simulink model "Algo_testing"  (R2017a)
settings: Solver=ode3  StartTime=0.0  StopTime=100  FixedStep=.01  RelTol=1e-3  EnableMultiTasking=on
undefined symbols (not defined in the file or in its folder): cap, soc
libraries: library x16, simulink x1
settings Model: SimulationMode=accelerator  Creator=Aniket Padghan  LastModifiedBy=Nagesh
settings DataIOCC: LimitDataPoints=on  SaveFormat=Array
settings OptimizationCC: LifeSpan=inf
settings DebuggingCC: SFUnexpectedBacktrackingDiag=warning  SFNoUnconditionalDefaultTransitionDiag=warning  SFExecutionAtInitializationDiag=none
settings HardwareCC: ProdBitPerPointer=32  ProdBitPerSizeT=32  ProdBitPerPtrDiffT=32  ProdLargestAtomicFloat=None  ProdIntDivRoundTo=Undefined  ProdEndianess=Unspecified  ProdWordSize=32  ProdHWDeviceType=32-bit Generic
settings ModelReferenceCC: PropagateSignalLabelsOutOfModel=off
settings GRTTargetCC: TargetLangStandard=C89/C90 (ANSI)  GeneratePreprocessorConditionals=Disable all
settings ConfigComp: CovMetricSettings=dw  CovHtmlReporting=on  CovSaveCumulativeToWorkspaceVar=on  CovSaveSingleToWorkspaceVar=on  CovExternalEMLEnable=off

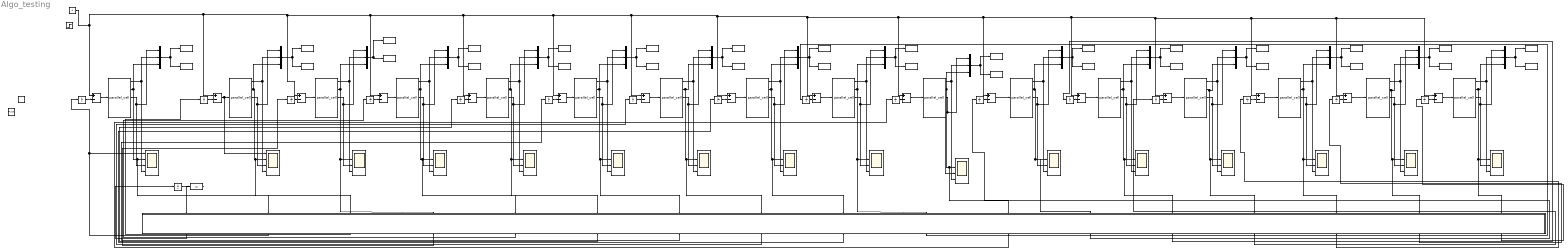
== system Algo_testing ==
  Constant : Constant  Value=-1
  IC : InitialCondition  Value=zeros(16,1)
  MATLAB Function : MATLAB Function  TreatAsAtomicUnit=on
  Mux{,1..15} (16 alike) : Mux  Inputs=3
  Pulse Generator : DiscretePulseGenerator  PulseType=Time based  Period=100  PulseWidth=50  SampleTime=0.01
  Repeating Sequence : simulink/Sources/Repeating Sequence  rep_seq_t=[0 50 100]  rep_seq_y=[0 1 0]
  Scope{,1..15} (16 alike) : Scope  NumInputPorts=4
  Step : Step  After=-1  SampleTime=0.01
  Subtract{,1,3..16} (16 alike) : Sum  Inputs=+-
  To Workspace : ToWorkspace  VariableName=VehicleBTimeSeries  SaveFormat=Timeseries  SampleTime=-1
      settings: Save2DSignal=2-D array (concatenate along first dimension)
  To Workspace1 : ToWorkspace  VariableName=VehicleBarray  SampleTime=-1
      settings: Save2DSignal=2-D array (concatenate along first dimension)
  To Workspace10 : ToWorkspace  VariableName=VehicleBTimeSeries5  SaveFormat=Timeseries  SampleTime=-1
      settings: Save2DSignal=2-D array (concatenate along first dimension)
  To Workspace11 : ToWorkspace  VariableName=VehicleBarray5  SampleTime=-1
      settings: Save2DSignal=2-D array (concatenate along first dimension)
  To Workspace12 : ToWorkspace  VariableName=VehicleBTimeSeries6  SaveFormat=Timeseries  SampleTime=-1
      settings: Save2DSignal=2-D array (concatenate along first dimension)
  To Workspace13 : ToWorkspace  VariableName=VehicleBarray6  SampleTime=-1
      settings: Save2DSignal=2-D array (concatenate along first dimension)
  To Workspace14 : ToWorkspace  VariableName=VehicleBTimeSeries7  SaveFormat=Timeseries  SampleTime=-1
      settings: Save2DSignal=2-D array (concatenate along first dimension)
  To Workspace15 : ToWorkspace  VariableName=VehicleBarray7  SampleTime=-1
      settings: Save2DSignal=2-D array (concatenate along first dimension)
  To Workspace16 : ToWorkspace  VariableName=VehicleBTimeSeries8  SaveFormat=Timeseries  SampleTime=-1
      settings: Save2DSignal=2-D array (concatenate along first dimension)
  To Workspace17 : ToWorkspace  VariableName=VehicleBarray8  SampleTime=-1
      settings: Save2DSignal=2-D array (concatenate along first dimension)
  To Workspace18 : ToWorkspace  VariableName=VehicleBTimeSeries9  SaveFormat=Timeseries  SampleTime=-1
      settings: Save2DSignal=2-D array (concatenate along first dimension)
  To Workspace19 : ToWorkspace  VariableName=VehicleBarray9  SampleTime=-1
      settings: Save2DSignal=2-D array (concatenate along first dimension)
  To Workspace2 : ToWorkspace  VariableName=VehicleBTimeSeries1  SaveFormat=Timeseries  SampleTime=-1
      settings: Save2DSignal=2-D array (concatenate along first dimension)
  To Workspace20 : ToWorkspace  VariableName=VehicleBTimeSeries10  SaveFormat=Timeseries  SampleTime=-1
      settings: Save2DSignal=2-D array (concatenate along first dimension)
  To Workspace21 : ToWorkspace  VariableName=VehicleBarray10  SampleTime=-1
      settings: Save2DSignal=2-D array (concatenate along first dimension)
  To Workspace22 : ToWorkspace  VariableName=VehicleBTimeSeries11  SaveFormat=Timeseries  SampleTime=-1
      settings: Save2DSignal=2-D array (concatenate along first dimension)
  To Workspace23 : ToWorkspace  VariableName=VehicleBarray11  SampleTime=-1
      settings: Save2DSignal=2-D array (concatenate along first dimension)
  To Workspace24 : ToWorkspace  VariableName=VehicleBTimeSeries12  SaveFormat=Timeseries  SampleTime=-1
      settings: Save2DSignal=2-D array (concatenate along first dimension)
  To Workspace25 : ToWorkspace  VariableName=VehicleBarray12  SampleTime=-1
      settings: Save2DSignal=2-D array (concatenate along first dimension)
  To Workspace26 : ToWorkspace  VariableName=VehicleBTimeSeries13  SaveFormat=Timeseries  SampleTime=-1
      settings: Save2DSignal=2-D array (concatenate along first dimension)
  To Workspace27 : ToWorkspace  VariableName=VehicleBarray13  SampleTime=-1
      settings: Save2DSignal=2-D array (concatenate along first dimension)
  To Workspace28 : ToWorkspace  VariableName=VehicleBTimeSeries14  SaveFormat=Timeseries  SampleTime=-1
      settings: Save2DSignal=2-D array (concatenate along first dimension)
  To Workspace29 : ToWorkspace  VariableName=VehicleBarray14  SampleTime=-1
      settings: Save2DSignal=2-D array (concatenate along first dimension)
  To Workspace3 : ToWorkspace  VariableName=VehicleBarray1  SampleTime=-1
      settings: Save2DSignal=2-D array (concatenate along first dimension)
  To Workspace30 : ToWorkspace  VariableName=VehicleBTimeSeries15  SaveFormat=Timeseries  SampleTime=-1
      settings: Save2DSignal=2-D array (concatenate along first dimension)
  To Workspace31 : ToWorkspace  VariableName=VehicleBarray15  SampleTime=-1
      settings: Save2DSignal=2-D array (concatenate along first dimension)
  To Workspace4 : ToWorkspace  VariableName=VehicleBTimeSeries2  SaveFormat=Timeseries  SampleTime=-1
      settings: Save2DSignal=2-D array (concatenate along first dimension)
  To Workspace5 : ToWorkspace  VariableName=VehicleBarray2  SampleTime=-1
      settings: Save2DSignal=2-D array (concatenate along first dimension)
  To Workspace6 : ToWorkspace  VariableName=VehicleBTimeSeries3  SaveFormat=Timeseries  SampleTime=-1
      settings: Save2DSignal=2-D array (concatenate along first dimension)
  To Workspace7 : ToWorkspace  VariableName=VehicleBarray3  SampleTime=-1
      settings: Save2DSignal=2-D array (concatenate along first dimension)
  To Workspace8 : ToWorkspace  VariableName=VehicleBTimeSeries4  SaveFormat=Timeseries  SampleTime=-1
      settings: Save2DSignal=2-D array (concatenate along first dimension)
  To Workspace9 : ToWorkspace  VariableName=VehicleBarray4  SampleTime=-1
      settings: Save2DSignal=2-D array (concatenate along first dimension)
  Unit Delay{,1..16} (17 alike) : UnitDelay  SampleTime=-1
  parallel_cell : library/parallel_cell  initial_SoC=soc(1)  cell_capacity=cap(1)  T_SoC_Breakpoints=T_SoC_Breakpoints  T_SoC_Table_Data=T_SoC_Table_Data  Rp_SoC_Table_Data=Rp_SoC_Table_Data  Rp_SoC_Breakpoints=Rp_SoC_Breakpoints  Ro_SoC_Table_Data=Ro_SoC_Table_Data  Ro_SoC_Breakpoints=Ro_SoC_Breakpoints  Em_SoC_Table_Data=Em_SoC_Table_Data  Em_SoC_Breakpoints=Em_SoC_Breakpoints
      link override Integrator: LowerSaturationLimit=-1*cell_capacity*3600
  parallel_cell1 : library/parallel_cell  initial_SoC=soc(2)  cell_capacity=cap(2)  T_SoC_Breakpoints=T_SoC_Breakpoints  T_SoC_Table_Data=T_SoC_Table_Data  Rp_SoC_Table_Data=Rp_SoC_Table_Data  Rp_SoC_Breakpoints=Rp_SoC_Breakpoints  Ro_SoC_Table_Data=Ro_SoC_Table_Data  Ro_SoC_Breakpoints=Ro_SoC_Breakpoints  Em_SoC_Table_Data=Em_SoC_Table_Data  Em_SoC_Breakpoints=Em_SoC_Breakpoints
      link override Integrator: LowerSaturationLimit=-1*cell_capacity*3600
  parallel_cell10 : library/parallel_cell  initial_SoC=soc(11)  cell_capacity=cap(11)  T_SoC_Breakpoints=T_SoC_Breakpoints  T_SoC_Table_Data=T_SoC_Table_Data  Rp_SoC_Table_Data=Rp_SoC_Table_Data  Rp_SoC_Breakpoints=Rp_SoC_Breakpoints  Ro_SoC_Table_Data=Ro_SoC_Table_Data  Ro_SoC_Breakpoints=Ro_SoC_Breakpoints  Em_SoC_Table_Data=Em_SoC_Table_Data  Em_SoC_Breakpoints=Em_SoC_Breakpoints
      link override Integrator: LowerSaturationLimit=-1*cell_capacity*3600
  parallel_cell11 : library/parallel_cell  initial_SoC=soc(12)  cell_capacity=cap(12)  T_SoC_Breakpoints=T_SoC_Breakpoints  T_SoC_Table_Data=T_SoC_Table_Data  Rp_SoC_Table_Data=Rp_SoC_Table_Data  Rp_SoC_Breakpoints=Rp_SoC_Breakpoints  Ro_SoC_Table_Data=Ro_SoC_Table_Data  Ro_SoC_Breakpoints=Ro_SoC_Breakpoints  Em_SoC_Table_Data=Em_SoC_Table_Data  Em_SoC_Breakpoints=Em_SoC_Breakpoints
      link override Integrator: LowerSaturationLimit=-1*cell_capacity*3600
  parallel_cell12 : library/parallel_cell  initial_SoC=soc(13)  cell_capacity=cap(13)  T_SoC_Breakpoints=T_SoC_Breakpoints  T_SoC_Table_Data=T_SoC_Table_Data  Rp_SoC_Table_Data=Rp_SoC_Table_Data  Rp_SoC_Breakpoints=Rp_SoC_Breakpoints  Ro_SoC_Table_Data=Ro_SoC_Table_Data  Ro_SoC_Breakpoints=Ro_SoC_Breakpoints  Em_SoC_Table_Data=Em_SoC_Table_Data  Em_SoC_Breakpoints=Em_SoC_Breakpoints
      link override Integrator: LowerSaturationLimit=-1*cell_capacity*3600
  parallel_cell13 : library/parallel_cell  initial_SoC=soc(14)  cell_capacity=cap(14)  T_SoC_Breakpoints=T_SoC_Breakpoints  T_SoC_Table_Data=T_SoC_Table_Data  Rp_SoC_Table_Data=Rp_SoC_Table_Data  Rp_SoC_Breakpoints=Rp_SoC_Breakpoints  Ro_SoC_Table_Data=Ro_SoC_Table_Data  Ro_SoC_Breakpoints=Ro_SoC_Breakpoints  Em_SoC_Table_Data=Em_SoC_Table_Data  Em_SoC_Breakpoints=Em_SoC_Breakpoints
      link override Integrator: LowerSaturationLimit=-1*cell_capacity*3600
  parallel_cell14 : library/parallel_cell  initial_SoC=soc(15)  cell_capacity=cap(15)  T_SoC_Breakpoints=T_SoC_Breakpoints  T_SoC_Table_Data=T_SoC_Table_Data  Rp_SoC_Table_Data=Rp_SoC_Table_Data  Rp_SoC_Breakpoints=Rp_SoC_Breakpoints  Ro_SoC_Table_Data=Ro_SoC_Table_Data  Ro_SoC_Breakpoints=Ro_SoC_Breakpoints  Em_SoC_Table_Data=Em_SoC_Table_Data  Em_SoC_Breakpoints=Em_SoC_Breakpoints
      link override Integrator: LowerSaturationLimit=-1*cell_capacity*3600
  parallel_cell15 : library/parallel_cell  initial_SoC=soc(16)  cell_capacity=cap(16)  T_SoC_Breakpoints=T_SoC_Breakpoints  T_SoC_Table_Data=T_SoC_Table_Data  Rp_SoC_Table_Data=Rp_SoC_Table_Data  Rp_SoC_Breakpoints=Rp_SoC_Breakpoints  Ro_SoC_Table_Data=Ro_SoC_Table_Data  Ro_SoC_Breakpoints=Ro_SoC_Breakpoints  Em_SoC_Table_Data=Em_SoC_Table_Data  Em_SoC_Breakpoints=Em_SoC_Breakpoints
      link override Integrator: LowerSaturationLimit=-1*cell_capacity*3600
  parallel_cell2 : library/parallel_cell  initial_SoC=soc(3)  cell_capacity=cap(3)  T_SoC_Breakpoints=T_SoC_Breakpoints  T_SoC_Table_Data=T_SoC_Table_Data  Rp_SoC_Table_Data=Rp_SoC_Table_Data  Rp_SoC_Breakpoints=Rp_SoC_Breakpoints  Ro_SoC_Table_Data=Ro_SoC_Table_Data  Ro_SoC_Breakpoints=Ro_SoC_Breakpoints  Em_SoC_Table_Data=Em_SoC_Table_Data  Em_SoC_Breakpoints=Em_SoC_Breakpoints
      link override Integrator: LowerSaturationLimit=-1*cell_capacity*3600
  parallel_cell3 : library/parallel_cell  initial_SoC=soc(4)  cell_capacity=cap(4)  T_SoC_Breakpoints=T_SoC_Breakpoints  T_SoC_Table_Data=T_SoC_Table_Data  Rp_SoC_Table_Data=Rp_SoC_Table_Data  Rp_SoC_Breakpoints=Rp_SoC_Breakpoints  Ro_SoC_Table_Data=Ro_SoC_Table_Data  Ro_SoC_Breakpoints=Ro_SoC_Breakpoints  Em_SoC_Table_Data=Em_SoC_Table_Data  Em_SoC_Breakpoints=Em_SoC_Breakpoints
      link override Integrator: LowerSaturationLimit=-1*cell_capacity*3600
  parallel_cell4 : library/parallel_cell  initial_SoC=soc(5)  cell_capacity=cap(5)  T_SoC_Breakpoints=T_SoC_Breakpoints  T_SoC_Table_Data=T_SoC_Table_Data  Rp_SoC_Table_Data=Rp_SoC_Table_Data  Rp_SoC_Breakpoints=Rp_SoC_Breakpoints  Ro_SoC_Table_Data=Ro_SoC_Table_Data  Ro_SoC_Breakpoints=Ro_SoC_Breakpoints  Em_SoC_Table_Data=Em_SoC_Table_Data  Em_SoC_Breakpoints=Em_SoC_Breakpoints
      link override Integrator: LowerSaturationLimit=-1*cell_capacity*3600
  parallel_cell5 : library/parallel_cell  initial_SoC=soc(6)  cell_capacity=cap(6)  T_SoC_Breakpoints=T_SoC_Breakpoints  T_SoC_Table_Data=T_SoC_Table_Data  Rp_SoC_Table_Data=Rp_SoC_Table_Data  Rp_SoC_Breakpoints=Rp_SoC_Breakpoints  Ro_SoC_Table_Data=Ro_SoC_Table_Data  Ro_SoC_Breakpoints=Ro_SoC_Breakpoints  Em_SoC_Table_Data=Em_SoC_Table_Data  Em_SoC_Breakpoints=Em_SoC_Breakpoints
      link override Integrator: LowerSaturationLimit=-1*cell_capacity*3600
  parallel_cell6 : library/parallel_cell  initial_SoC=soc(7)  cell_capacity=cap(7)  T_SoC_Breakpoints=T_SoC_Breakpoints  T_SoC_Table_Data=T_SoC_Table_Data  Rp_SoC_Table_Data=Rp_SoC_Table_Data  Rp_SoC_Breakpoints=Rp_SoC_Breakpoints  Ro_SoC_Table_Data=Ro_SoC_Table_Data  Ro_SoC_Breakpoints=Ro_SoC_Breakpoints  Em_SoC_Table_Data=Em_SoC_Table_Data  Em_SoC_Breakpoints=Em_SoC_Breakpoints
      link override Integrator: LowerSaturationLimit=-1*cell_capacity*3600
  parallel_cell7 : library/parallel_cell  initial_SoC=soc(8)  cell_capacity=cap(8)  T_SoC_Breakpoints=T_SoC_Breakpoints  T_SoC_Table_Data=T_SoC_Table_Data  Rp_SoC_Table_Data=Rp_SoC_Table_Data  Rp_SoC_Breakpoints=Rp_SoC_Breakpoints  Ro_SoC_Table_Data=Ro_SoC_Table_Data  Ro_SoC_Breakpoints=Ro_SoC_Breakpoints  Em_SoC_Table_Data=Em_SoC_Table_Data  Em_SoC_Breakpoints=Em_SoC_Breakpoints
      link override Integrator: LowerSaturationLimit=-1*cell_capacity*3600
  parallel_cell8 : library/parallel_cell  initial_SoC=soc(9)  cell_capacity=cap(9)  T_SoC_Breakpoints=T_SoC_Breakpoints  T_SoC_Table_Data=T_SoC_Table_Data  Rp_SoC_Table_Data=Rp_SoC_Table_Data  Rp_SoC_Breakpoints=Rp_SoC_Breakpoints  Ro_SoC_Table_Data=Ro_SoC_Table_Data  Ro_SoC_Breakpoints=Ro_SoC_Breakpoints  Em_SoC_Table_Data=Em_SoC_Table_Data  Em_SoC_Breakpoints=Em_SoC_Breakpoints
      link override Integrator: LowerSaturationLimit=-1*cell_capacity*3600
  parallel_cell9 : library/parallel_cell  initial_SoC=soc(10)  cell_capacity=cap(10)  T_SoC_Breakpoints=T_SoC_Breakpoints  T_SoC_Table_Data=T_SoC_Table_Data  Rp_SoC_Table_Data=Rp_SoC_Table_Data  Rp_SoC_Breakpoints=Rp_SoC_Breakpoints  Ro_SoC_Table_Data=Ro_SoC_Table_Data  Ro_SoC_Breakpoints=Ro_SoC_Breakpoints  Em_SoC_Table_Data=Em_SoC_Table_Data  Em_SoC_Breakpoints=Em_SoC_Breakpoints
      link override Integrator: LowerSaturationLimit=-1*cell_capacity*3600
  wires:
  parallel_cell/1 -> Scope/4, Mux/2
  Mux/1 -> To Workspace/1, To Workspace1/1
  parallel_cell/2 -> Mux/3, MATLAB Function/2(v1), Scope/2
  parallel_cell/3 -> Mux/1, Scope/3
  parallel_cell1/1 -> Scope1/4, Mux1/2
  parallel_cell1/2 -> Mux1/3, MATLAB Function/3(v2), Scope1/2
  Mux1/1 -> To Workspace2/1, To Workspace3/1
  parallel_cell1/3 -> Mux1/1, Scope1/3
  parallel_cell2/1 -> Scope2/4, Mux2/2
  parallel_cell2/2 -> Mux2/3, MATLAB Function/4(v3), Scope2/2
  Mux2/1 -> To Workspace5/1, To Workspace4/1
  parallel_cell2/3 -> Mux2/1, Scope2/3
  parallel_cell3/1 -> Scope3/4, Mux3/2
  parallel_cell3/2 -> Mux3/3, MATLAB Function/5(v4), Scope3/2
  Mux3/1 -> To Workspace6/1, To Workspace7/1
  parallel_cell3/3 -> Mux3/1, Scope3/3
  parallel_cell4/1 -> Scope4/4, Mux4/2
  parallel_cell4/2 -> Mux4/3, MATLAB Function/6(v5), Scope4/2
  Mux4/1 -> To Workspace8/1, To Workspace9/1
  parallel_cell4/3 -> Mux4/1, Scope4/3
  parallel_cell5/1 -> Scope5/4, Mux5/2
  parallel_cell5/2 -> Mux5/3, MATLAB Function/7(v6), Scope5/2
  Mux5/1 -> To Workspace10/1, To Workspace11/1
  parallel_cell5/3 -> Mux5/1, Scope5/3
  parallel_cell6/1 -> Scope6/4, Mux6/2
  parallel_cell6/2 -> Mux6/3, MATLAB Function/8(v7), Scope6/2
  Mux6/1 -> To Workspace12/1, To Workspace13/1
  parallel_cell11/2 -> Mux11/3, MATLAB Function/13(v12), Scope11/2
  parallel_cell11/1 -> Scope11/4, Mux11/2
  parallel_cell7/1 -> Scope7/4, Mux7/2
  parallel_cell10/3 -> Mux10/1, Scope10/3
  parallel_cell6/3 -> Mux6/1, Scope6/3
  Mux11/1 -> To Workspace14/1, To Workspace15/1
  parallel_cell7/2 -> Mux7/3, MATLAB Function/9(v8), Scope7/2
  parallel_cell10/2 -> Mux10/3, MATLAB Function/12(v11), Scope10/2
  Mux10/1 -> To Workspace24/1, To Workspace25/1
  parallel_cell9/3 -> Scope9/3, Mux9/1
  parallel_cell8/2 -> Mux8/3, MATLAB Function/10(v9), Scope8/2
  Mux9/1 -> To Workspace22/1, To Workspace23/1
  Mux7/1 -> To Workspace18/1, To Workspace19/1
  parallel_cell9/1 -> Scope9/4, Mux9/2
  parallel_cell8/3 -> Mux8/1, Scope8/3
  parallel_cell10/1 -> Scope10/4, Mux10/2
  parallel_cell7/3 -> Mux7/1, Scope7/3
  Mux12/1 -> To Workspace16/1, To Workspace17/1
  parallel_cell12/2 -> Mux12/3, MATLAB Function/14(v13), Scope12/2
  parallel_cell8/1 -> Scope8/4, Mux8/2
  Mux8/1 -> To Workspace20/1, To Workspace21/1
  parallel_cell12/1 -> Scope12/4, Mux12/2
  parallel_cell11/3 -> Mux11/1, Scope11/3
  parallel_cell9/2 -> Mux9/3, MATLAB Function/11(v10), Scope9/2
  parallel_cell15/2 -> Mux15/3, MATLAB Function/17(v16), Scope15/2
  Mux15/1 -> To Workspace28/1, To Workspace29/1
  parallel_cell12/3 -> Mux12/1, Scope12/3
  Mux13/1 -> To Workspace30/1, To Workspace31/1
  parallel_cell15/1 -> Scope15/4, Mux15/2
  parallel_cell14/3 -> Mux14/1, Scope14/3
  parallel_cell15/3 -> Mux15/1, Scope15/3
  parallel_cell13/2 -> Mux13/3, MATLAB Function/15(v14), Scope13/2
  Mux14/1 -> To Workspace26/1, To Workspace27/1
  parallel_cell14/2 -> Mux14/3, MATLAB Function/16(v15), Scope14/2
  parallel_cell14/1 -> Scope14/4, Mux14/2
  parallel_cell13/1 -> Scope13/4, Mux13/2
  parallel_cell13/3 -> Mux13/1, Scope13/3
  Subtract/1 -> parallel_cell/1
  Subtract15/1 -> parallel_cell15/1
  Subtract1/1 -> Scope1/1, parallel_cell1/1
  Subtract3/1 -> parallel_cell3/1
  Subtract4/1 -> parallel_cell4/1
  Subtract5/1 -> parallel_cell5/1
  Subtract6/1 -> parallel_cell6/1
  Subtract7/1 -> parallel_cell7/1
  Subtract8/1 -> parallel_cell8/1
  Subtract9/1 -> parallel_cell9/1
  Subtract10/1 -> parallel_cell10/1
  Subtract11/1 -> parallel_cell11/1
  Subtract12/1 -> parallel_cell12/1
  Subtract13/1 -> parallel_cell13/1
  Subtract14/1 -> parallel_cell14/1
  MATLAB Function/2(i1) -> Scope/1, Unit Delay/1
  MATLAB Function/3(i2) -> Unit Delay1/1
  MATLAB Function/5(i4) -> Unit Delay3/1
  MATLAB Function/6(i5) -> Unit Delay4/1
  MATLAB Function/7(i6) -> Unit Delay5/1
  MATLAB Function/8(i7) -> Unit Delay6/1
  MATLAB Function/9(i8) -> Unit Delay7/1
  MATLAB Function/10(i9) -> Unit Delay8/1
  MATLAB Function/11(i10) -> Unit Delay9/1
  MATLAB Function/12(i11) -> Unit Delay10/1
  MATLAB Function/13(i12) -> Unit Delay11/1
  MATLAB Function/14(i13) -> Unit Delay12/1
  MATLAB Function/15(i14) -> Unit Delay13/1
  MATLAB Function/16(i15) -> Unit Delay14/1
  MATLAB Function/17(i16) -> Unit Delay15/1
  Constant/1 -> Subtract16/1, Subtract15/1, Subtract14/1, Subtract13/1, Subtract12/1, Subtract11/1, Subtract10/1, Subtract9/1, Subtract8/1, Subtract7/1, Subtract6/1, Subtract5/1, Subtract4/1, Subtract3/1, Subtract1/1, Subtract/1
  Unit Delay/1 -> Subtract/2
  Unit Delay1/1 -> Subtract1/2
  Unit Delay2/1 -> Subtract16/2
  Subtract16/1 -> parallel_cell2/1
  Unit Delay3/1 -> Subtract3/2
  Unit Delay4/1 -> Subtract4/2
  Unit Delay5/1 -> Subtract5/2
  Unit Delay6/1 -> Subtract6/2
  Unit Delay7/1 -> Subtract7/2
  Unit Delay8/1 -> Subtract8/2
  Unit Delay9/1 -> Subtract9/2
  Unit Delay10/1 -> Subtract10/2
  Unit Delay11/1 -> Subtract11/2
  Unit Delay12/1 -> Subtract12/2
  Unit Delay13/1 -> Subtract13/2
  Unit Delay14/1 -> Subtract14/2
  Unit Delay15/1 -> Subtract15/2
  MATLAB Function/4(i3) -> Unit Delay2/1
  IC/1 -> MATLAB Function/1("vlast ")
  MATLAB Function/1(vlast) -> Unit Delay16/1
  Unit Delay16/1 -> IC/1

== matlab function Algo_testing/MATLAB Function ==
  data: vlast output; vlast input; v1 input; i1 output; v2 input; v3 input; v4 input; v5 input; v6 input; v7 input; v8 input; v9 input; v10 input; v11 input; v12 input; v13 input; v14 input; v15 input; v16 input; i2 output; i3 output; i4 output; i5 output; i6 output; i7 output; i8 output; i9 output; i10 output; i11 output; i12 output; i13 output; i14 output; i15 output; i16 output
function [vlast, i1,i2,i3,i4,i5,i6,i7,i8,i9,i10,i11,i12,i13,i14,i15,i16] = fcn(vlast,v1,v2,v3,v4,v5,v6,v7,v8,v9,v10,v11,v12,v13,v14,v15,v16)
v=zeros(16,1);
v(1)=v1;v(2)=v2;v(3)=v3;v(4)=v4;v(5)=v5;v(6)=v6;v(7)=v7;v(8)=v8;
v(9)=v9;v(10)=v10;v(11)=v11;v(12)=v12;v(13)=v13;v(14)=v14;v(15)=v15;v(16)=v16;

i=zeros(16,1);

%identify the best
% % vdelmin=min(v-vlast);
% % vmin=min(v);
% % 
% % score=zeros(16,1);
% % for j=1:16
% %     if(v(j)-vlast(j)==vdelmin)
% %         score(j)=score(j)+1;
% %         if(v(j)==vmin)
% %             score(j)=score(j)+1;
% %         end
% %     end
% % end
% % 
% % bestid = find(score==2,1);
% % if(bestid==0)
% %     bestid = find(score==1,1);
% % end

vmod=v;
bestid=11;
%switching_control
for j=1:16
    vmod(j)=(0.2*v(j)+0.8*vlast(j));
end

DSGCURRENT=-0.1;
windowmargin=0.01;
for j=1:16
    if(vmod(j)-vmod(bestid)>windowmargin)
    i(j)=DSGCURRENT;
    end
end

for j=1:16
    if(v(j)==3.82)
        i=-1*ones(1*16);
end

vlast=v;
%create vlast in adv

i1=i(1);i2=i(2);i3=i(3);i4=i(4);i5=i(5);i6=i(6);i7=i(7);i8=i(8);
i9=i(9);i10=i(10);i11=i(11);i12=i(12);i13=i(13);i14=i(14);i15=i(15);i16=i(16);
